simulink model "train"  (R2012b)
settings: Solver=ode45  StartTime=0.0  StopTime=10.0  RelTol=1e-3
settings Model: Creator=fofo  LastModifiedBy=fofo

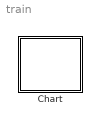
== system train ==
  Chart : Stateflow chart  TreatAsAtomicUnit=on

== stateflow chart train/Chart ==
  state Train0
    state urgent_inc
      du:
      distance_dot=dir*v;
      v_dot=0.5;
      distance_out[i]=distance;
    state recover
      du:distance_dot=dir*v;
      v_dot=-0.5;
      distance_out[i]=distance;
    state urgent_stop
      du:distance_dot=0;
      v_dot=0;distance_out[i]=distance;
      ex:maxv=sqrt(0.5*abs(S[j]-distance))
    state init
      du:time_dot=1;
    state urgent_dec
      du:
      distance_dot=dir*v;
      v_dot=-1.5;
      distance_out[i]=distance;
    state near
      du:
      distance_dot=dir*v;
      v_dot=acc;
      distance_out[i]=distance;
    state stop
      en:v=0;
    state tmp
    state stablerun
      du:
      distance_dot=dir*v;
      v_dot=0;
      distance_out[i]=distance;
    state run
      en:j=j+dir;
      du:distance_dot=dir*v;
      v_dot=0.5;
      distance_out[i]=distance;
    state ChangeDirection
      du:time_dot=1;
    (default) -> init : {i=0,start[i]=0,stop[i]=0,
        | time=0,distance=0,
        | v=0,dir=1;}
    urgent_inc -> recover [order 1] : [v==maxv]
    urgent_stop -> urgent_inc : [urstart[i]==1]
    recover -> (junction 10) [order 1] : [urstop[i]==1]
    recover -> stop [order 2] : [abs(distance-S[j])<=1&& v==0]{stop[i]=1}
    urgent_inc -> (junction 10) [order 2] : [urstop[i]==1]
    urgent_dec -> urgent_stop : [v==0]
    (junction 10) -> urgent_dec
    init -> stop : [time>=Delay[i]]{stop[i]=1,j=0;}
    near -> stop [order 1] : [abs(distance-S[j])<=1&&v<=0.5]
        | {stop[i]=1,start[i]=0;}
    near -> urgent_dec [order 2] : [urstop[i]==1]
    stop -> tmp : [start[i]==1]
        | {stop[i]=0,time=0;}
    ChangeDirection -> stop : [time>=30]
        | {dir=-dir,
        | stop[i]=1,
        | start[i]=0;}
    run -> urgent_dec [order 3] : [urstop[i]==1]
    stablerun -> urgent_dec [order 2] : [urstop[i]==1]
    (junction 11) -> near : {acc=-v^2*0.001}
    tmp -> run [order 3] : [(dir==1&&j<N-1)||(dir==-1&&j>0)]
    tmp -> ChangeDirection [order 1] : [j==0&&dir==-1]
    tmp -> ChangeDirection [order 2] : [j==N-1&&dir==1]
    stablerun -> (junction 11) [order 1] : [abs(distance-S[j])<=500]
    run -> (junction 11) [order 1] : [abs(distance-S[j])<=500]
    run -> stablerun [order 2] : [v>=20]
  data: v local double; j local double; dir local int32 =1; maxv local double; time local double; i local int32; distance local double; acc local double
  data v settings: updateMethod=SF_CONTINUOUS_TIME_DATA
  data time settings: updateMethod=SF_CONTINUOUS_TIME_DATA
  data distance settings: updateMethod=SF_CONTINUOUS_TIME_DATA
